simulink model "LQI_Metodo_Simulink"  (R2022a)
settings: Solver=VariableStepAuto  StartTime=0.0  StopTime=10  RelTol=1e-3
undefined symbols (not defined in the file): A, B, C, Kei, Kf, Kf_t, Ki, Kr
settings Model: Creator=gabri  LastModifiedBy=gabri

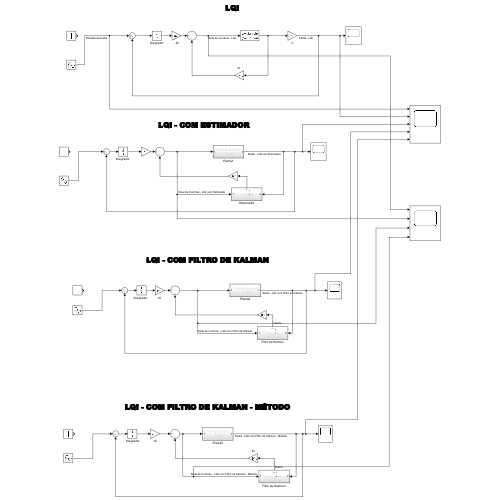
[thumbnail: Simulink's stored preview of the top-level diagram]
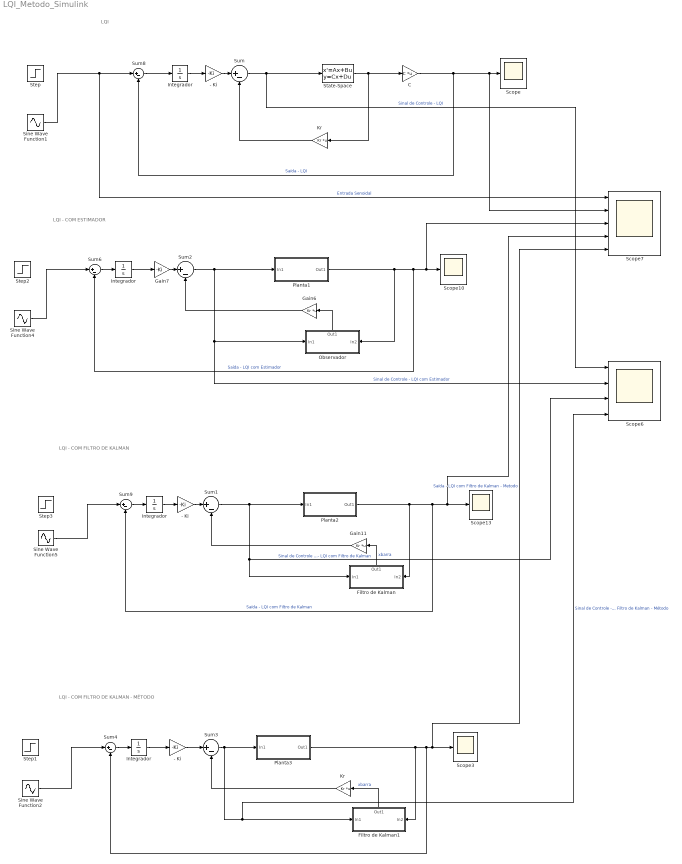
== system LQI_Metodo_Simulink ==
  note: LQI
  note: LQI - COM ESTIMADOR
  note: LQI - COM FILTRO DE KALMAN
  note: LQI - COM FILTRO DE KALMAN - MÉTODO
  " Integrador" : Integrator
  " Kr" : Gain  Gain=Kr  Multiplication=Matrix(K*u)
  - Ki : Gain  Gain=-Ki
  "- Ki " : Gain  Gain=-Ki
  "- Ki  " : Gain  Gain=-Ki
  C : Gain  Gain=C  Multiplication=Matrix(K*u)
  Filtro de Kalman : Subsystem
      settings: PortSchema="{\"entries\":[{\"content\":{\"sides\":[{\"content\":{\"connectorIds\":[\"In1\"]},\"type\":\"ConnectorPlacement.EquallySpacedRectSide\",\"uuid\":\"a39a08db-6117-4f96-90c3-02f1f7ffb9ec\"},{\"content\":{\"connectorIds\":[\"In2\"],\"side\":\"RIGHT\"},\"type\":\"ConnectorPlacement.EquallySpacedRectSide\",\"uuid\":\"e0a0a54b-1f6f-4425-9f49-01d22204810c\"},{\"content\":{\"connectorIds\":[\"Out1\"],\"side\":\"TOP\"},\"type\":\"ConnectorPlacement.EquallySpacedRectSide\",\"uuid\":\"f9c2d93e-7541-4a9e-b077-600f0b58f20b\"},{\"content\":{\"connectorIds\":[],\"side\":\"BOTTOM\"},\"type\":\"ConnectorPlacement.EquallySpacedRectSide\",\"uuid\":\"2e0212ac-38a2-465c-9330-e4bad70b5dfc\"}]},\"type\":\"ConnectorPlacement.EquallySpacedConnector\",\"uuid\":\"106c2d4c-b59c-4d15-84b9-899fdea4a460\"}],\"packageUris\":[\"http://schema.mathworks.com/mf0/Connector/R2020b\"],\"version\":\"1.0\"}"
  Filtro de Kalman1 : Subsystem
      settings: PortSchema="{\"entries\":[{\"content\":{\"sides\":[{\"content\":{\"connectorIds\":[\"In1\"]},\"type\":\"ConnectorPlacement.EquallySpacedRectSide\",\"uuid\":\"a39a08db-6117-4f96-90c3-02f1f7ffb9ec\"},{\"content\":{\"connectorIds\":[\"In2\"],\"side\":\"RIGHT\"},\"type\":\"ConnectorPlacement.EquallySpacedRectSide\",\"uuid\":\"e0a0a54b-1f6f-4425-9f49-01d22204810c\"},{\"content\":{\"connectorIds\":[\"Out1\"],\"side\":\"TOP\"},\"type\":\"ConnectorPlacement.EquallySpacedRectSide\",\"uuid\":\"f9c2d93e-7541-4a9e-b077-600f0b58f20b\"},{\"content\":{\"connectorIds\":[],\"side\":\"BOTTOM\"},\"type\":\"ConnectorPlacement.EquallySpacedRectSide\",\"uuid\":\"2e0212ac-38a2-465c-9330-e4bad70b5dfc\"}]},\"type\":\"ConnectorPlacement.EquallySpacedConnector\",\"uuid\":\"106c2d4c-b59c-4d15-84b9-899fdea4a460\"}],\"packageUris\":[\"http://schema.mathworks.com/mf0/Connector/R2020b\"],\"version\":\"1.0\"}"
  Gain11 : Gain  Gain=Kr  Multiplication=Matrix(K*u)
  Gain6 : Gain  Gain=Kr  Multiplication=Matrix(K*u)
  Gain7 : Gain  Gain=-Ki
  Integrador : Integrator
  "Integrador " : Integrator
  "Integrador  " : Integrator
  Kr : Gain  Gain=Kr  Multiplication=Matrix(K*u)
  Observador : Subsystem
      settings: PortSchema="{\"entries\":[{\"content\":{\"sides\":[{\"content\":{\"connectorIds\":[\"In1\"]},\"type\":\"ConnectorPlacement.EquallySpacedRectSide\",\"uuid\":\"a39a08db-6117-4f96-90c3-02f1f7ffb9ec\"},{\"content\":{\"connectorIds\":[\"In2\"],\"side\":\"RIGHT\"},\"type\":\"ConnectorPlacement.EquallySpacedRectSide\",\"uuid\":\"e0a0a54b-1f6f-4425-9f49-01d22204810c\"},{\"content\":{\"connectorIds\":[\"Out1\"],\"side\":\"TOP\"},\"type\":\"ConnectorPlacement.EquallySpacedRectSide\",\"uuid\":\"f9c2d93e-7541-4a9e-b077-600f0b58f20b\"},{\"content\":{\"connectorIds\":[],\"side\":\"BOTTOM\"},\"type\":\"ConnectorPlacement.EquallySpacedRectSide\",\"uuid\":\"2e0212ac-38a2-465c-9330-e4bad70b5dfc\"}]},\"type\":\"ConnectorPlacement.EquallySpacedConnector\",\"uuid\":\"106c2d4c-b59c-4d15-84b9-899fdea4a460\"}],\"packageUris\":[\"http://schema.mathworks.com/mf0/Connector/R2020b\"],\"version\":\"1.0\"}"
  Planta1 : Subsystem
  Planta2 : Subsystem
  Planta3 : Subsystem
  Scope{,3,10,13} (4 alike) : Scope
  Scope6 : Scope  NumInputPorts=4
  Scope7 : Scope  NumInputPorts=5
  Sine Wave Function{1..2,4..5} (4 alike) : Sin  Amplitude=0.001  Frequency=pi  SampleTime=0
  State-Space : StateSpace  A=A  B=B  C=eye(3)  D=[0;0;0]  InitialCondition=0
  Step{,1..3} (4 alike) : Step  Time=0  After=0.002  SampleTime=0
  Sum{,1..4,6,8..9} (8 alike) : Sum  Inputs=|+-
  wires:
  State-Space/1 -> Kr/1, C/1
  C/1 -> Scope7/2, Scope/1, Sum8/2  "Saída - LQI"
  Kr/1 -> Sum/2
  Gain7/1 -> Sum2/1
  Sum2/1 -> Scope6/2, Observador/1(In1), Planta1/1(In1)  "Sinal de Controle - LQI com Estimador"
  Observador/1(Out1) -> Gain6/1
  "Integrador "/1 -> Gain7/1
  Gain6/1 -> Sum2/2
  Planta1/1(Out1) -> Sum6/2, Scope7/3, Scope10/1, Observador/2(In2)  "Saída - LQI com Estimador"
  Sum9/1 -> "Integrador  "/1
  Gain11/1 -> Sum1/2
  "- Ki  "/1 -> Sum1/1
  Planta2/1(Out1) -> Filtro de Kalman/2(In2), Sum9/2, Scope7/4, Scope13/1  "Saída - LQI com Filtro de Kalman"
  Sum1/1 -> Filtro de Kalman/1(In1), Scope6/3, Planta2/1(In1)  "Sinal de Controle - LQI com Filtro de Kalman"
  Filtro de Kalman/1(Out1) -> Gain11/1  "xbarra"
  "Integrador  "/1 -> "- Ki  "/1
  Sum/1 -> Scope6/1, State-Space/1  "Sinal de Controle - LQI"
  Sum6/1 -> "Integrador "/1
  Sum8/1 -> Integrador/1
  Integrador/1 -> - Ki/1
  - Ki/1 -> Sum/1
  Sum4/1 -> " Integrador"/1
  Sum3/1 -> Planta3/1(In1), Scope6/4, Filtro de Kalman1/1(In1)  "Sinal de Controle - LQI com Filtro de Kalman - Método"
  Filtro de Kalman1/1(Out1) -> " Kr"/1  "xbarra"
  " Integrador"/1 -> "- Ki "/1
  " Kr"/1 -> Sum3/2
  Planta3/1(Out1) -> Filtro de Kalman1/2(In2), Sum4/2, Scope7/5, Scope3/1  "Saída - LQI com Filtro de Kalman - Metodo"
  "- Ki "/1 -> Sum3/1
  Sine Wave Function1/1 -> Scope7/1, Sum8/1  "Entrada Senoidal"
  Sine Wave Function5/1 -> Sum9/1
  Sine Wave Function2/1 -> Sum4/1
  Sine Wave Function4/1 -> Sum6/1

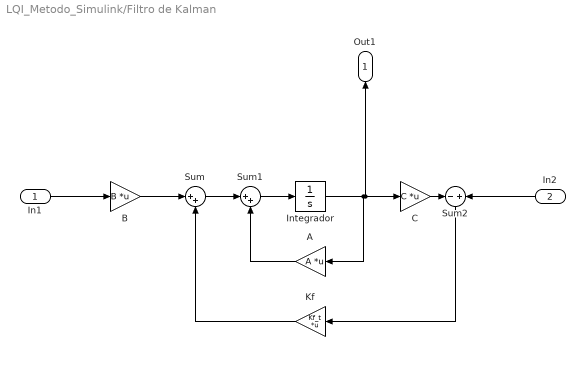
== system LQI_Metodo_Simulink/Filtro de Kalman ==
  In1 : Inport
  In2 : Inport  Port=2
  A : Gain  Gain=A  Multiplication=Matrix(K*u)
  B : Gain  Gain=B  Multiplication=Matrix(K*u)
  C : Gain  Gain=C  Multiplication=Matrix(K*u)
  Integrador : Integrator
  Kf : Gain  Gain=Kf_t  Multiplication=Matrix(K*u)
  Sum : Sum  Inputs=|++
  Sum1 : Sum  Inputs=|++
  Sum2 : Sum  Inputs=-|+
  Out1 : Outport
  wires:
  In1/1 -> B/1
  B/1 -> Sum/1
  Sum/1 -> Sum1/1
  Sum1/1 -> Integrador/1
  Integrador/1 -> Out1/1, C/1, A/1
  C/1 -> Sum2/1
  In2/1 -> Sum2/2
  Sum2/1 -> Kf/1
  Kf/1 -> Sum/2
  A/1 -> Sum1/2

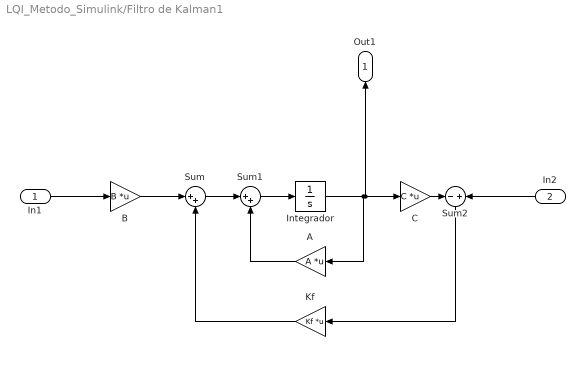
== system LQI_Metodo_Simulink/Filtro de Kalman1 ==
  In1 : Inport
  In2 : Inport  Port=2
  A : Gain  Gain=A  Multiplication=Matrix(K*u)
  B : Gain  Gain=B  Multiplication=Matrix(K*u)
  C : Gain  Gain=C  Multiplication=Matrix(K*u)
  Integrador : Integrator
  Kf : Gain  Gain=Kf  Multiplication=Matrix(K*u)
  Sum : Sum  Inputs=|++
  Sum1 : Sum  Inputs=|++
  Sum2 : Sum  Inputs=-|+
  Out1 : Outport
  wires:
  In1/1 -> B/1
  B/1 -> Sum/1
  Sum/1 -> Sum1/1
  Sum1/1 -> Integrador/1
  Integrador/1 -> Out1/1, C/1, A/1
  C/1 -> Sum2/1
  In2/1 -> Sum2/2
  Sum2/1 -> Kf/1
  Kf/1 -> Sum/2
  A/1 -> Sum1/2

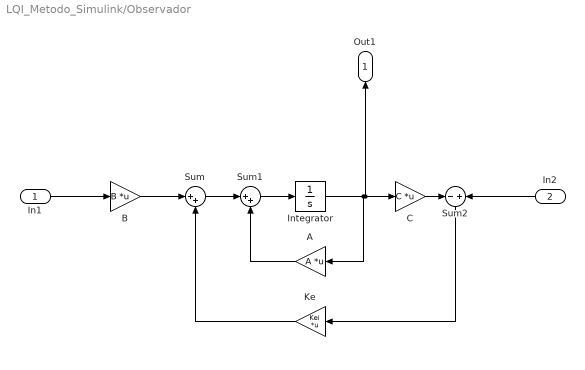
== system LQI_Metodo_Simulink/Observador ==
  In1 : Inport
  In2 : Inport  Port=2
  A : Gain  Gain=A  Multiplication=Matrix(K*u)
  B : Gain  Gain=B  Multiplication=Matrix(K*u)
  C : Gain  Gain=C  Multiplication=Matrix(K*u)
  Integrator : Integrator
  Ke : Gain  Gain=Kei  Multiplication=Matrix(K*u)
  Sum : Sum  Inputs=|++
  Sum1 : Sum  Inputs=|++
  Sum2 : Sum  Inputs=-|+
  Out1 : Outport
  wires:
  In1/1 -> B/1
  B/1 -> Sum/1
  Sum/1 -> Sum1/1
  Sum1/1 -> Integrator/1
  Integrator/1 -> C/1, Out1/1, A/1
  C/1 -> Sum2/1
  In2/1 -> Sum2/2
  Sum2/1 -> Ke/1
  Ke/1 -> Sum/2
  A/1 -> Sum1/2

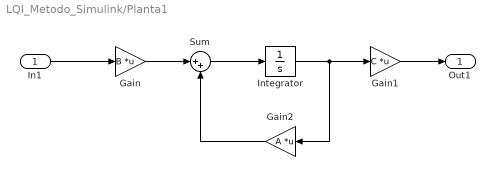
== system LQI_Metodo_Simulink/Planta1 ==
  In1 : Inport
  Gain : Gain  Gain=B  Multiplication=Matrix(K*u)
  Gain1 : Gain  Gain=C  Multiplication=Matrix(K*u)
  Gain2 : Gain  Gain=A  Multiplication=Matrix(K*u)
  Integrator : Integrator
  Sum : Sum  Inputs=|++
  Out1 : Outport
  wires:
  In1/1 -> Gain/1
  Gain/1 -> Sum/1
  Sum/1 -> Integrator/1
  Integrator/1 -> Gain2/1, Gain1/1
  Gain1/1 -> Out1/1
  Gain2/1 -> Sum/2

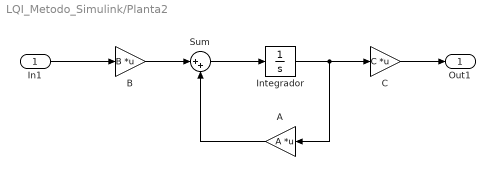
== system LQI_Metodo_Simulink/Planta2 ==
  In1 : Inport
  A : Gain  Gain=A  Multiplication=Matrix(K*u)
  B : Gain  Gain=B  Multiplication=Matrix(K*u)
  C : Gain  Gain=C  Multiplication=Matrix(K*u)
  Integrador : Integrator
  Sum : Sum  Inputs=|++
  Out1 : Outport
  wires:
  In1/1 -> B/1
  B/1 -> Sum/1
  Sum/1 -> Integrador/1
  Integrador/1 -> C/1, A/1
  A/1 -> Sum/2
  C/1 -> Out1/1

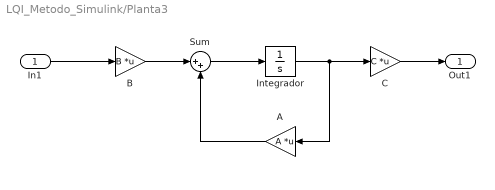
== system LQI_Metodo_Simulink/Planta3 ==
  In1 : Inport
  A : Gain  Gain=A  Multiplication=Matrix(K*u)
  B : Gain  Gain=B  Multiplication=Matrix(K*u)
  C : Gain  Gain=C  Multiplication=Matrix(K*u)
  Integrador : Integrator
  Sum : Sum  Inputs=|++
  Out1 : Outport
  wires:
  In1/1 -> B/1
  B/1 -> Sum/1
  Sum/1 -> Integrador/1
  Integrador/1 -> C/1, A/1
  A/1 -> Sum/2
  C/1 -> Out1/1
